simulink model "Comp_MCU_main"  (R2024a)
settings: Solver=FixedStepDiscrete  StartTime=0.0  StopTime=10.0  RelTol=1e-3  EnableMultiTasking=on
settings Model: DataDictionary=APPTypes.sldd  Creator=FVT23010  LastModifiedBy=FVT23010
settings SolverCC: AutoInsertRateTranBlk=on
settings DataIOCC: SaveFormat=StructureWithTime
settings OptimizationCC: DefaultParameterBehavior=Inlined  EnhancedBackFolding=on  PassReuseOutputArgsAs=Individual arguments  ZeroExternalMemoryAtStartup=off  ZeroInternalMemoryAtStartup=off  OptimizeBlockOrder=speed  DifferentSizesBufferReuse=on  OptimizationCustomize=off  EfficientTunableParamExpr=on
settings DebuggingCC: ParameterTunabilityLossMsg=error
settings ModelReferenceCC: ModelReferenceNumInstancesAllowed=Single
settings SFSimCC: MATLABDynamicMemAlloc=off
settings RTWCC: Description=AUTOSAR  SystemTargetFile=autosar.tlc  GenCodeOnly=on  TemplateMakefile=ert_default_tmf  DataTypeReplacement=CDataTypesFixedWidth
settings CodeAppCC: ForceParamTrailComments=on  IgnoreCustomStorageClasses=off  OperatorAnnotations=on  SimulinkDataObjDesc=on  SFDataObjDesc=on  InsertBlockDesc=on
settings STFCustomTargetCC: MultiwordLength=256  ParMdlRefBuildCompliant=on  CompOptLevelCompliant=on  IncludeMdlTerminateFcn=off  CombineOutputUpdateFcns=on  SuppressErrorStatus=on  ERTCustomFileBanners=on  SupportNonFinite=off  SupportComplex=off  SupportContinuousTime=off  SupportNonInlinedSFcns=off  RemoveResetFunc=on  MATLABClassNameForMDSCustomization=Simulink.SoftwareTarget.ERTCustomization  AutosarCompliant=on  GRTInterface=off  LookupTableObjectStructAxisOrder=2,1,3,4,...  LUTObjectStructOrderEvenSpacing=Size,Table,Breakpoints  SystemTargetFile=autosar.tlc
settings ERTTargetCC: TargetLangStandard=C99 (ISO)  ConcurrentExecutionCompliant=off  IncludeMdlTerminateFcn=off  SuppressErrorStatus=on  SupportNonFinite=off  SupportComplex=off  ModelStepFunctionPrototypeControlCompliant=off  CPPClassGenCompliant=off  AutosarCompliant=on  LookupTableObjectStructAxisOrder=2,1,3,4,...  LUTObjectStructOrderEvenSpacing=Size,Table,Breakpoints  InlinedParameterPlacement=NonHierarchical  ERTCustomFileTemplate=example_file_process.tlc  BooleanTrueId=TRUE  BooleanFalseId=FALSE

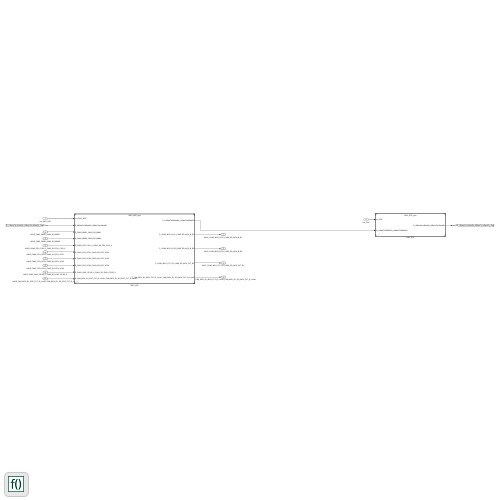
[thumbnail: Simulink's stored preview of the top-level diagram]
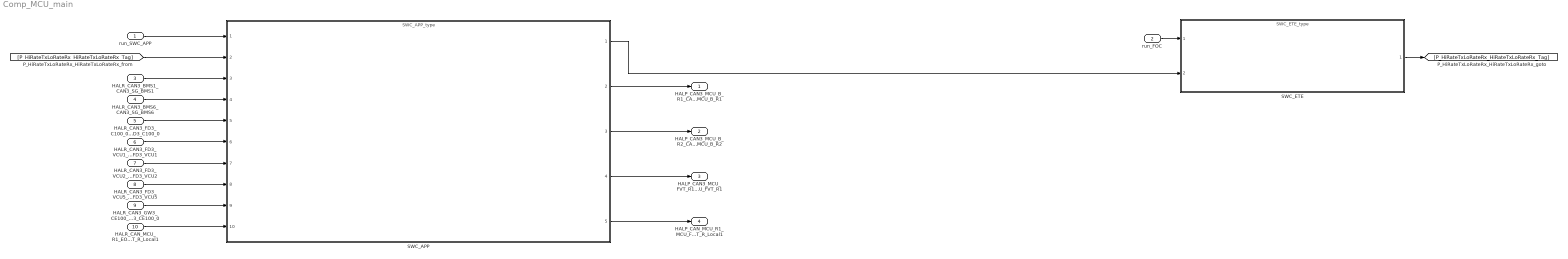
== system Comp_MCU_main ==
  run_SWC_APP : Inport  SampleTime=0.001  OutputFunctionCall=on
  run_FOC : Inport  Port=2  OutputFunctionCall=on
  HALR_CAN3_BMS1_CAN3_SG_BMS1 : Inport  Port=3  OutDataTypeStr=Bus: DT_CAN3_SG_BMS1  PortDimensions=1  BusOutputAsStruct=on
  HALR_CAN3_BMS6_CAN3_SG_BMS6 : Inport  Port=4  OutDataTypeStr=Bus: DT_CAN3_SG_BMS6  PortDimensions=1  BusOutputAsStruct=on
  HALR_CAN3_FD3_C100_0_CAN3_SG_FD3_C100_0 : Inport  Port=5  OutDataTypeStr=Bus: DT_CAN3_SG_FD3_C100_0  PortDimensions=1  BusOutputAsStruct=on
  HALR_CAN3_FD3_VCU1_CAN3_SG_FD3_VCU1 : Inport  Port=6  OutDataTypeStr=Bus: DT_CAN3_SG_FD3_VCU1  PortDimensions=1  BusOutputAsStruct=on
  HALR_CAN3_FD3_VCU2_CAN3_SG_FD3_VCU2 : Inport  Port=7  OutDataTypeStr=Bus: DT_CAN3_SG_FD3_VCU2  PortDimensions=1  BusOutputAsStruct=on
  HALR_CAN3_FD3_VCU5_CAN3_SG_FD3_VCU5 : Inport  Port=8  OutDataTypeStr=Bus: DT_CAN3_SG_FD3_VCU5  PortDimensions=1  BusOutputAsStruct=on
  HALR_CAN3_GW3_CE100_0_CAN3_SG_GW3_CE100_0 : Inport  Port=9  OutDataTypeStr=Bus: DT_CAN3_SG_GW3_CE100_0  PortDimensions=1  BusOutputAsStruct=on
  HALR_CAN_MCU_R1_EOP_FVT_R_Local1_CAN_MCU_R1_SG_EOP_FVT_R_Local1 : Inport  Port=10  OutDataTypeStr=Bus: DT_CAN_MCU_R1_SG_EOP_FVT_R_Local1  PortDimensions=1  BusOutputAsStruct=on
  SWC_APP : ModelReference  ModelNameDialog=SWC_APP_type  SimulationMode=Normal  ScheduleRates=on  ModelReferenceVersion=1.1
  SWC_ETE : ModelReference  ModelNameDialog=SWC_ETE_type  SimulationMode=Normal  ScheduleRates=on  ModelReferenceVersion=1.1
  HALP_CAN3_MCU_B_R1_CAN3_SG_MCU_B_R1 : Outport  OutDataTypeStr=Bus: DT_CAN3_SG_MCU_B_R1  PortDimensions=1  BusOutputAsStruct=on
  HALP_CAN3_MCU_B_R2_CAN3_SG_MCU_B_R2 : Outport  Port=2  OutDataTypeStr=Bus: DT_CAN3_SG_MCU_B_R2  PortDimensions=1  BusOutputAsStruct=on
  HALP_CAN3_MCU_FVT_R1_CAN3_SG_MCU_FVT_R1 : Outport  Port=3  OutDataTypeStr=Bus: DT_CAN3_SG_MCU_FVT_R1  PortDimensions=1  BusOutputAsStruct=on
  HALP_CAN_MCU_R1_MCU_FVT_R_Local1_CAN_MCU_R1_SG_MCU_FVT_R_Local1 : Outport  Port=4  OutDataTypeStr=Bus: DT_CAN_MCU_R1_SG_MCU_FVT_R_Local1  PortDimensions=1  BusOutputAsStruct=on
  wires:
  run_SWC_APP/1 -> SWC_APP/1
  run_FOC/1 -> SWC_ETE/1
  HALR_CAN3_BMS1_CAN3_SG_BMS1/1 -> SWC_APP/3
  HALR_CAN3_BMS6_CAN3_SG_BMS6/1 -> SWC_APP/4
  HALR_CAN3_FD3_C100_0_CAN3_SG_FD3_C100_0/1 -> SWC_APP/5
  HALR_CAN3_FD3_VCU1_CAN3_SG_FD3_VCU1/1 -> SWC_APP/6
  HALR_CAN3_FD3_VCU2_CAN3_SG_FD3_VCU2/1 -> SWC_APP/7
  HALR_CAN3_FD3_VCU5_CAN3_SG_FD3_VCU5/1 -> SWC_APP/8
  HALR_CAN3_GW3_CE100_0_CAN3_SG_GW3_CE100_0/1 -> SWC_APP/9
  HALR_CAN_MCU_R1_EOP_FVT_R_Local1_CAN_MCU_R1_SG_EOP_FVT_R_Local1/1 -> SWC_APP/10
  SWC_APP/2 -> HALP_CAN3_MCU_B_R1_CAN3_SG_MCU_B_R1/1
  SWC_APP/3 -> HALP_CAN3_MCU_B_R2_CAN3_SG_MCU_B_R2/1
  SWC_APP/4 -> HALP_CAN3_MCU_FVT_R1_CAN3_SG_MCU_FVT_R1/1
  SWC_APP/5 -> HALP_CAN_MCU_R1_MCU_FVT_R_Local1_CAN_MCU_R1_SG_MCU_FVT_R_Local1/1
  SWC_APP/1 -> SWC_ETE/2
  SWC_ETE/1 -> [P_HiRateTxLoRateRx_HiRateTxLoRateRx_Tag]
  [P_HiRateTxLoRateRx_HiRateTxLoRateRx_Tag] -> SWC_APP/2
